simulink model "JenaFox_NCm"  (R2018a)
settings: Solver=ode23s  StartTime=0.0  StopTime=20  MaxStep=maxStep  RelTol=1e-3  AbsTol=absTol
values from neighbouring files (symbols this model uses):
  amplifier = 2.28    [init_motor_parameters.m]
  c_coupling_hip = 7/hip_Ra*hip_k/hip_i    (= 1.22844788155)    [init_motor_parameters.m]
  c_coupling_knee = 7/knee_Ra*knee_k/knee_i    (= 0.698088436179)    [init_motor_parameters.m]
  c_hs = 0.1    [Fox_param.m]
  d_coupling_knee = 0.5    [init_motor_parameters.m]
  d_hs = 0.35    [Fox_param.m]
  g = 9.80665    [Fox_param.m]    (also in init_motor_parameters.m = 9.81)
  hip_i = 1/300.4858    (= 0.00332794428223)    [init_motor_parameters.m]
  hip_Jm = 1/2*hip_m*hip_r^2    (= 1e-07)    [init_motor_parameters.m]
  hip_k = (hip_Um-hip_I0*hip_Ra)*60/(2*pi*hip_n0)    (= 0.00320895298542)    [init_motor_parameters.m]
  hip_Mrg = hip_k*hip_I0g    (= 0.000320895298542)    [init_motor_parameters.m]
  hip_Mrhg = hip_k*hip_Iag    (= 0.000381865405265)    [init_motor_parameters.m]
  hip_na = (hip_Us-(hip_I0*hip_Ra))/hip_k    (= 105.13168591)    [init_motor_parameters.m]
  hip_Ra = hip_Um/hip_Is    (= 5.49450549451)    [init_motor_parameters.m]
  IC_motor_hip_l = deg2rad(IC_phi_hip_l/hip_i)    [init_motor_parameters.m]
  IC_motor_hip_r = deg2rad(IC_phi_hip_r/hip_i)    [init_motor_parameters.m]
  IC_motor_knee_l = deg2rad(IC_phi_knee_l/knee_i)    [init_motor_parameters.m]
  IC_motor_knee_r = deg2rad(IC_phi_knee_r/knee_i)    [init_motor_parameters.m]
  IC_phi_hip_l = 10    [Fox_param.m]
  IC_phi_hip_r = -29    [Fox_param.m]
  IC_v_motor_hip = 0    [init_motor_parameters.m]
  IC_v_motor_knee = 0    [init_motor_parameters.m]
  k_gx = 10*M_RB/0.01    [Fox_param.m]
  k_gy = 150*M_RB/0.01    [Fox_param.m]
  knee_i = 1/185.8428    (= 0.00538089180748)    [init_motor_parameters.m]
  knee_Jm = 1/2*knee_m*knee_r^2    (= 3.2e-08)    [init_motor_parameters.m]
  knee_k = (knee_Um-knee_I0*knee_Ra)*60/(2*pi*knee_n0)    (= 0.000596244182085)    [init_motor_parameters.m]
  knee_Mrg = knee_k*knee_I0g    (= 6.55868600293e-05)    [init_motor_parameters.m]
  knee_Mrhg = knee_k*knee_Iag    (= 9.59953133156e-05)    [init_motor_parameters.m]
  knee_na = (knee_Us-knee_I0*knee_Ra)/knee_k    (= 1360.36733855)    [init_motor_parameters.m]
  knee_Ra = knee_Um/knee_Is    (= 1.11111111111)    [init_motor_parameters.m]
  mu_slide = 4.6    [Fox_param.m]
  mu_stick = 0.8    [Fox_param.m]
  v_gx_max = 0.06    [Fox_param.m]
  v_gy_max = 0.70    (= 0.7)    [Fox_param.m]
  vLimit = 0.01    [Fox_param.m]
undefined symbols (not defined in the file or in its folder): param, smiData, X, Y, Z
libraries: sm_lib x38, nesl_utility x32, simulink x22, simulink_extras x8
(part 3 of 3)

== system JenaFox_NCm/Subsystem/Ground Contact Model/Ground Friction Model/X-Axis Kinetic Friction Model ==
  note: Kinetic Friction Model
  note: Footpoint Determiner
  note: Sliding Limit Detector
  pos [m] : Inport
  vel [m/s] : Inport  Port=2
  F_Normal [N] : Inport  Port=3
  Enable : EnablePort  StatesWhenEnabling=reset  PropagateVarSize=During execution
  Abs : Abs
  Constant : Constant  Value=vLimit
  FixPt Relational Operator : RelationalOperator  Operator=>  OutDataTypeStr=boolean  ZeroCross=off  RndMeth=Nearest
  Memory : Memory  InheritSampleTime=on
  Negative : simulink/Logic and Bit Operations/Compare To Zero  relop=<  OutDataTypeStr=boolean
  Product : Product  RndMeth=Zero
  Sign1 : Signum
  Sum : Sum  Inputs=|+-
  reverse : Gain  Gain=-1
  sliding friction coefficient : Gain  Gain=mu_slide
  posFP [m] : Outport
      settings: AttributesFormatString=initial = '%<InitialOutput>'\nwhen disabled = '%<OutputWhenDisabled>'
  Stiction! : Outport  Port=2  OutputWhenDisabled=reset  InitialOutput=0
      settings: AttributesFormatString=initial = '%<InitialOutput>'\nwhen disabled = '%<OutputWhenDisabled>'
  F_Slide [N] : Outport  Port=3  OutputWhenDisabled=reset  InitialOutput=0
      settings: AttributesFormatString=initial = '%<InitialOutput>'\nwhen disabled = '%<OutputWhenDisabled>'
  wires:
  reverse/1 -> Product/1
  F_Normal [N]/1 -> sliding friction coefficient/1
  vel [m/s]/1 -> Sign1/1, Abs/1
  pos [m]/1 -> posFP [m]/1
  Product/1 -> F_Slide [N]/1
  sliding friction coefficient/1 -> Product/2
  Sign1/1 -> reverse/1
  Memory/1 -> FixPt Relational Operator/2
  Negative/1 -> Memory/1, FixPt Relational Operator/1
  Abs/1 -> Sum/1
  Sum/1 -> Negative/1
  Constant/1 -> Sum/2
  FixPt Relational Operator/1 -> Stiction!/1

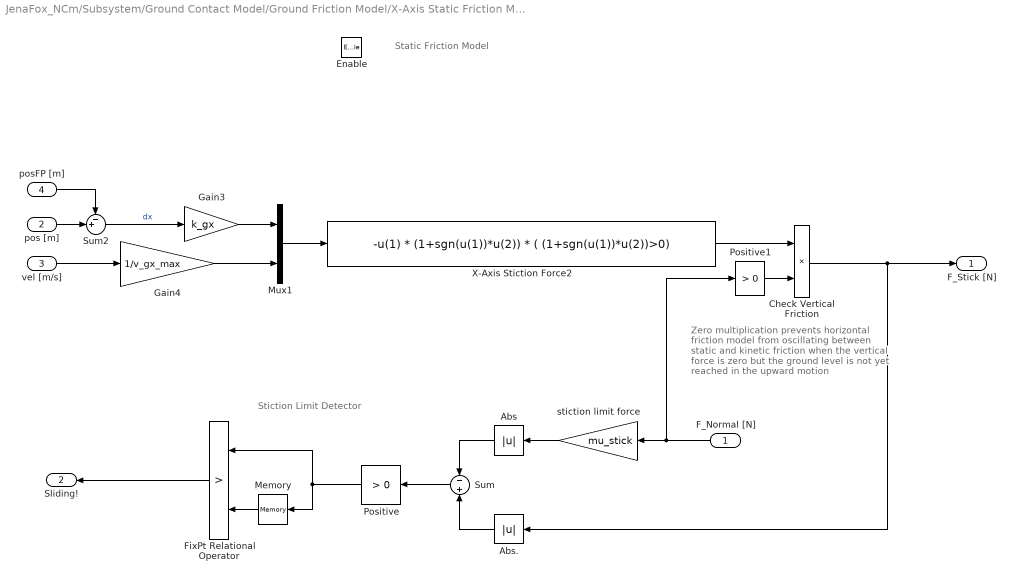
== system JenaFox_NCm/Subsystem/Ground Contact Model/Ground Friction Model/X-Axis Static Friction Model ==
  note: Stiction Limit Detector
  note: Static Friction Model
  note: Zero multiplication prevents
      | horizontal friction model from
      | oscillating between static and kinetic
      | friction when the vertical force is zero but
      | the ground level is not yet reached
      | in the upward motion
  F_Normal [N] : Inport
  pos [m] : Inport  Port=2
  vel [m/s] : Inport  Port=3
  posFP [m] : Inport  Port=4
  Enable : EnablePort  StatesWhenEnabling=reset  PropagateVarSize=During execution
  Abs : Abs
  Abs. : Abs
  Check Vertical Friction : Product  RndMeth=Zero
  FixPt Relational Operator : RelationalOperator  Operator=>  OutDataTypeStr=boolean  ZeroCross=off  RndMeth=Nearest
  Gain3 : Gain  Gain=k_gx
  Gain4 : Gain  Gain=1/v_gx_max
  Memory : Memory
  Mux1 : Mux  Inputs=2
  Positive : simulink/Logic and Bit Operations/Compare To Zero  relop=>  OutDataTypeStr=boolean
  Positive1 : simulink/Logic and Bit Operations/Compare To Zero  relop=>  OutDataTypeStr=boolean
  Sum : Sum  Inputs=-+
  Sum2 : Sum  Inputs=-+|
  X-Axis Stiction Force2 : Fcn  Expr=-u(1) * (1+sgn(u(1))*u(2)) * ( (1+sgn(u(1))*u(2))>0)
  stiction limit force : Gain  Gain=mu_stick
  F_Stick [N] : Outport  OutputWhenDisabled=reset  InitialOutput=0
      settings: AttributesFormatString=when disabled: %<OutputWhenDisabled>\ninitial: %<InitialOutput>
  Sliding! : Outport  Port=2  OutputWhenDisabled=reset  InitialOutput=0
      settings: AttributesFormatString=when disabled: %<OutputWhenDisabled>\ninitial: %<InitialOutput>
  wires:
  F_Normal [N]/1 -> stiction limit force/1, Positive1/1
  Sum2/1 -> Gain3/1  "dx"
  pos [m]/1 -> Sum2/2
  posFP [m]/1 -> Sum2/1
  vel [m/s]/1 -> Gain4/1
  Sum/1 -> Positive/1
  Memory/1 -> FixPt Relational Operator/2
  Positive/1 -> FixPt Relational Operator/1, Memory/1
  Abs./1 -> Sum/2
  Mux1/1 -> X-Axis Stiction Force2/1
  Gain3/1 -> Mux1/1
  Gain4/1 -> Mux1/2
  FixPt Relational Operator/1 -> Sliding!/1
  Abs/1 -> Sum/1
  stiction limit force/1 -> Abs/1
  Positive1/1 -> Check Vertical Friction/2
  Check Vertical Friction/1 -> F_Stick [N]/1, Abs./1
  X-Axis Stiction Force2/1 -> Check Vertical Friction/1

== system JenaFox_NCm/Subsystem/Ground Contact Model1/Ground Friction Model/Friction Switch ==
  note: Static/Kinetic Friction Switch
  Slide! : Inport
  Stick! : Inport  Port=2
  Memory : Memory
  S-R Flip-Flop : simulink_extras/Flip Flops/S-R Flip-Flop  initial_condition=1
  Terminator : Terminator
  Stiction : Outport
  wires:
  S-R Flip-Flop/1 -> Memory/1
  S-R Flip-Flop/2 -> Terminator/1
  Stick!/1 -> S-R Flip-Flop/1
  Slide!/1 -> S-R Flip-Flop/2
  Memory/1 -> Stiction/1

== system JenaFox_NCm/Subsystem/Ground Contact Model1/Ground Friction Model/X-Axis Kinetic Friction Model ==
  note: Kinetic Friction Model
  note: Footpoint Determiner
  note: Sliding Limit Detector
  pos [m] : Inport
  vel [m/s] : Inport  Port=2
  F_Normal [N] : Inport  Port=3
  Enable : EnablePort  StatesWhenEnabling=reset  PropagateVarSize=During execution
  Abs : Abs
  Constant : Constant  Value=vLimit
  FixPt Relational Operator : RelationalOperator  Operator=>  OutDataTypeStr=boolean  ZeroCross=off  RndMeth=Nearest
  Memory : Memory  InheritSampleTime=on
  Negative : simulink/Logic and Bit Operations/Compare To Zero  relop=<  OutDataTypeStr=boolean
  Product : Product  RndMeth=Zero
  Sign1 : Signum
  Sum : Sum  Inputs=|+-
  reverse : Gain  Gain=-1
  sliding friction coefficient : Gain  Gain=mu_slide
  posFP [m] : Outport
      settings: AttributesFormatString=initial = '%<InitialOutput>'\nwhen disabled = '%<OutputWhenDisabled>'
  Stiction! : Outport  Port=2  OutputWhenDisabled=reset  InitialOutput=0
      settings: AttributesFormatString=initial = '%<InitialOutput>'\nwhen disabled = '%<OutputWhenDisabled>'
  F_Slide [N] : Outport  Port=3  OutputWhenDisabled=reset  InitialOutput=0
      settings: AttributesFormatString=initial = '%<InitialOutput>'\nwhen disabled = '%<OutputWhenDisabled>'
  wires:
  reverse/1 -> Product/1
  F_Normal [N]/1 -> sliding friction coefficient/1
  vel [m/s]/1 -> Sign1/1, Abs/1
  pos [m]/1 -> posFP [m]/1
  Product/1 -> F_Slide [N]/1
  sliding friction coefficient/1 -> Product/2
  Sign1/1 -> reverse/1
  Memory/1 -> FixPt Relational Operator/2
  Negative/1 -> Memory/1, FixPt Relational Operator/1
  Abs/1 -> Sum/1
  Sum/1 -> Negative/1
  Constant/1 -> Sum/2
  FixPt Relational Operator/1 -> Stiction!/1

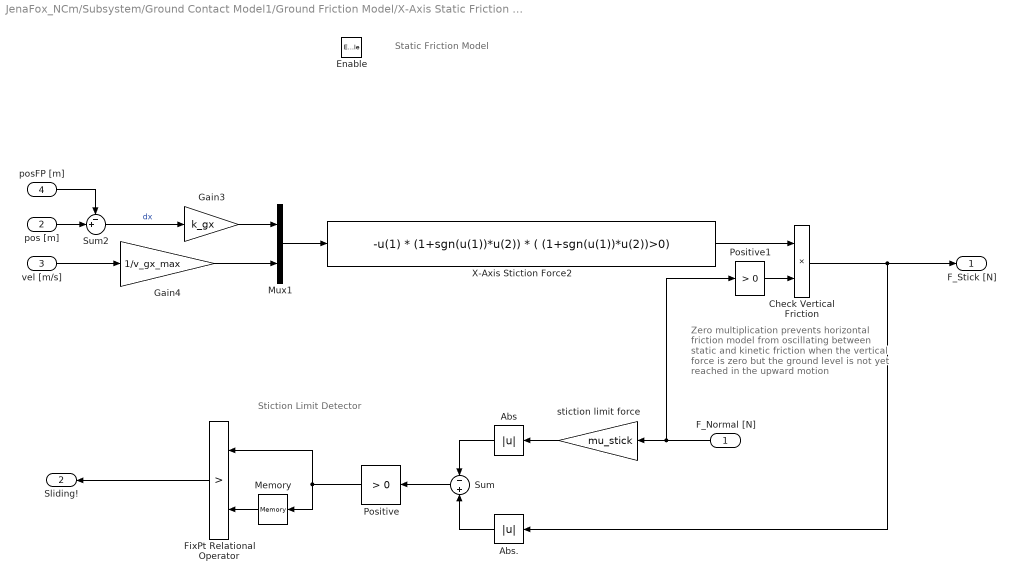
== system JenaFox_NCm/Subsystem/Ground Contact Model1/Ground Friction Model/X-Axis Static Friction Model ==
  note: Stiction Limit Detector
  note: Static Friction Model
  note: Zero multiplication prevents
      | horizontal friction model from
      | oscillating between static and kinetic
      | friction when the vertical force is zero but
      | the ground level is not yet reached
      | in the upward motion
  F_Normal [N] : Inport
  pos [m] : Inport  Port=2
  vel [m/s] : Inport  Port=3
  posFP [m] : Inport  Port=4
  Enable : EnablePort  StatesWhenEnabling=reset  PropagateVarSize=During execution
  Abs : Abs
  Abs. : Abs
  Check Vertical Friction : Product  RndMeth=Zero
  FixPt Relational Operator : RelationalOperator  Operator=>  OutDataTypeStr=boolean  ZeroCross=off  RndMeth=Nearest
  Gain3 : Gain  Gain=k_gx
  Gain4 : Gain  Gain=1/v_gx_max
  Memory : Memory
  Mux1 : Mux  Inputs=2
  Positive : simulink/Logic and Bit Operations/Compare To Zero  relop=>  OutDataTypeStr=boolean
  Positive1 : simulink/Logic and Bit Operations/Compare To Zero  relop=>  OutDataTypeStr=boolean
  Sum : Sum  Inputs=-+
  Sum2 : Sum  Inputs=-+|
  X-Axis Stiction Force2 : Fcn  Expr=-u(1) * (1+sgn(u(1))*u(2)) * ( (1+sgn(u(1))*u(2))>0)
  stiction limit force : Gain  Gain=mu_stick
  F_Stick [N] : Outport  OutputWhenDisabled=reset  InitialOutput=0
      settings: AttributesFormatString=when disabled: %<OutputWhenDisabled>\ninitial: %<InitialOutput>
  Sliding! : Outport  Port=2  OutputWhenDisabled=reset  InitialOutput=0
      settings: AttributesFormatString=when disabled: %<OutputWhenDisabled>\ninitial: %<InitialOutput>
  wires:
  F_Normal [N]/1 -> stiction limit force/1, Positive1/1
  Sum2/1 -> Gain3/1  "dx"
  pos [m]/1 -> Sum2/2
  posFP [m]/1 -> Sum2/1
  vel [m/s]/1 -> Gain4/1
  Sum/1 -> Positive/1
  Memory/1 -> FixPt Relational Operator/2
  Positive/1 -> FixPt Relational Operator/1, Memory/1
  Abs./1 -> Sum/2
  Mux1/1 -> X-Axis Stiction Force2/1
  Gain3/1 -> Mux1/1
  Gain4/1 -> Mux1/2
  FixPt Relational Operator/1 -> Sliding!/1
  Abs/1 -> Sum/1
  stiction limit force/1 -> Abs/1
  Positive1/1 -> Check Vertical Friction/2
  Check Vertical Friction/1 -> F_Stick [N]/1, Abs./1
  X-Axis Stiction Force2/1 -> Check Vertical Friction/1

== system JenaFox_NCm/Subsystem/simulation terminator/Subsystem/Subsystem ==
  In1 : Inport
  Enable : EnablePort  StatesWhenEnabling=reset
  Compare To Constant5 : simulink/Logic and Bit Operations/Compare To Constant  relop=>=  const=5  OutDataTypeStr=boolean
  Out1 : Outport
  wires:
  Compare To Constant5/1 -> Out1/1
  In1/1 -> Compare To Constant5/1

== matlab function JenaFox_NCm/joint torque calculation ==
  data: t input; U output; phi input; GC input; y_old input; y_old output; param input
function [U,y_old] = neural_controller(t,phi,GC,y_old,param)

%% controller settings
phi = phi';

t_old = y_old(1,1);
yFh_old = y_old(2,:);
yEh_old = y_old(3,:);
yFk_old = y_old(4,:);
yEk_old = y_old(5,:);

tau = 0.01;    %[s] time constant
alpha = 2;     %[1] response constant
Phi_Eh = param(1); %5;  %[deg] threshold sensor neuron hip extension, figure 5
Phi_Fh = param(2); %-10; %[deg] threshold sensor neuron hip flexion
Phi_AL = Phi_Fh;
Phi_AR = Phi_Fh;
Phi_Ek = -3;
Phi_Fk = -80;
Phi_GL = 0.2;
Phi_GR = 0.2;
Phi_M = 1;    %bias firing treshold
M_Amp = 3;
GM_h = param(3); %1.5;
GM_k = 0.9 * GM_h;
s_emh = 1;
s_fmh = -1;
s_emk = 1;
s_fmk = -1;

%% sensor neurons

%hip stretch receptors AL/AR, indicates when AEA is reached (hip flexed)
rho_AL = neuron(alpha,phi(2),Phi_AL);
rho_AR = neuron(alpha,phi(1),Phi_AR);

%ground contact sensors
rho_GL = neuron(alpha,Phi_GL,GC(2)-GC(1));
rho_GR = neuron(alpha,Phi_GR,GC(1)-GC(2));

% joint angle sensors hip
rho_Eh = neuron(alpha,Phi_Eh,phi(1:2));
rho_Fh = neuron(alpha,phi(1:2),Phi_Fh);

% joint angle sensors knee
rho_Ek = neuron(alpha,Phi_Ek,phi(3:4));
rho_Fk = neuron(alpha,phi(3:4),Phi_Fk);

%% motor neurons

%hip motor neurons
yEh = yEh_old * exp(-(t-t_old)/tau) + (-30) .* rho_Eh + [10 -10] .* rho_GR + [-10 10] .* rho_GL;
yFh = yFh_old * exp(-(t-t_old)/tau) + (-30) .* rho_Fh + [-10 10] .* rho_GR + [10 -10] .* rho_GL;

uEh = 1./(1 + exp(Phi_M-yEh));
uFh = 1./(1 + exp(Phi_M-yFh));

%knee motor neurons
yEk = yEk_old * exp(-(t-t_old)/tau) + (-30) .* rho_Ek + 15 .* [rho_AR rho_AL] + [10 -10] .* rho_GR + [-10 10] .* rho_GL;
yFk = yFk_old * exp(-(t-t_old)/tau) + (-30) .* rho_Fk + (-15) .* [rho_AR rho_AL] + [-10 10] .* rho_GR + [10 -10] .* rho_GL;

uEk = 1./(1 + exp(Phi_M-yEk));
uFk = 1./(1 + exp(Phi_M-yFk));

U = [M_Amp * GM_h .* (s_emh .* uEh + s_fmh .* uFh), M_Amp * GM_k .* (s_emk .* uEk + s_fmk .* uFk)]';

y_old(1,:) = [t 0];
y_old(3,:) = yEh;
y_old(2,:) = yFh;
y_old(5,:) = yEk;
y_old(4,:) = yFk;

    function rho = neuron(alpha,Phi_d,phi)
        rho = 1./(1 + exp(alpha .* (Phi_d - phi)));
    end

end
